simulink model "steering_mpc"  (R2024b)
settings: Solver=VariableStepAuto  StartTime=0  StopTime=84  FixedStep=0.001  RelTol=1e-3  AbsTol=1e-6
values from neighbouring files (symbols this model uses):
  m = 1575    [model.m]
undefined symbols (not defined in the file or in its folder): h, km, MPCController, s, sigbuilder_block
libraries: simulink_extras x6, ctrlSharedLib x2, aerolibconvert2 x2, Solver_SF x1, slpidlib x1
settings Model: Creator=dhall  LastModifiedBy=yassine
settings SolverCC: AlgebraicLoopSolver=TrustRegion
settings DataIOCC: SaveFormat=Array  SignalLoggingSaveFormat=ModelDataLogs  ReturnWorkspaceOutputs=off  SignalLoggingName=sigsOut
settings OptimizationCC: BooleanDataType=off  ReuseModelBlockBuffer=off  InitFltsAndDblsToZero=on
settings DebuggingCC: SaveWithParameterizedLinksMsg=none  UnderspecifiedInitializationDetection=Classic  MergeDetectMultiDrivingBlocksExec=none  SignalResolutionControl=TryResolveAllWithWarning  MultiTaskDSMMsg=warning  MultiTaskCondExecSysMsg=none  UnconnectedInputMsg=warning  UnconnectedOutputMsg=warning  UnconnectedLineMsg=warning
settings HardwareCC: ProdBitPerPointer=32  ProdBitPerSizeT=32  ProdBitPerPtrDiffT=32  ProdLargestAtomicFloat=None  ProdIntDivRoundTo=Undefined  ProdEndianess=Unspecified  ProdWordSize=32  ProdHWDeviceType=32-bit Generic  TargetUnknown=on
settings ModelReferenceCC: EnableRefExpFcnMdlSchedulingChecks=on  PropagateSignalLabelsOutOfModel=off
settings RTWCC: TemplateMakefile=grt_vc.tmf  GPUComputeCapability=3.5  DLArmComputeVersion=19.05
settings GRTTargetCC: TargetFcnLib=ansi_tfl_tmw.mat  TargetLangStandard=C89/C90 (ANSI)  ModelReferenceCompliant=off  CombineOutputUpdateFcns=off  MatFileLogging=off  GRTInterface=on
settings ConfigComp: CovMetricSettings=dw  CovSaveCumulativeToWorkspaceVar=on  CovSaveSingleToWorkspaceVar=on

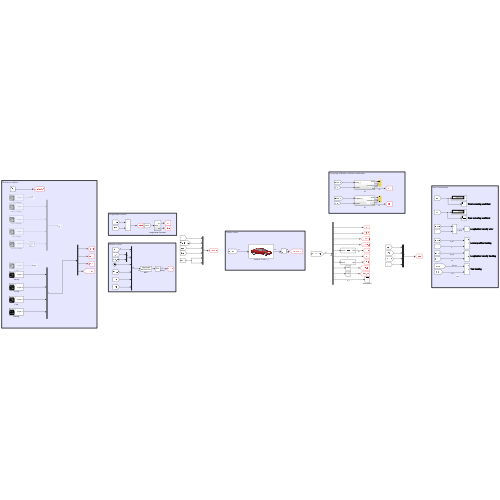
[thumbnail: Simulink's stored preview of the top-level diagram]
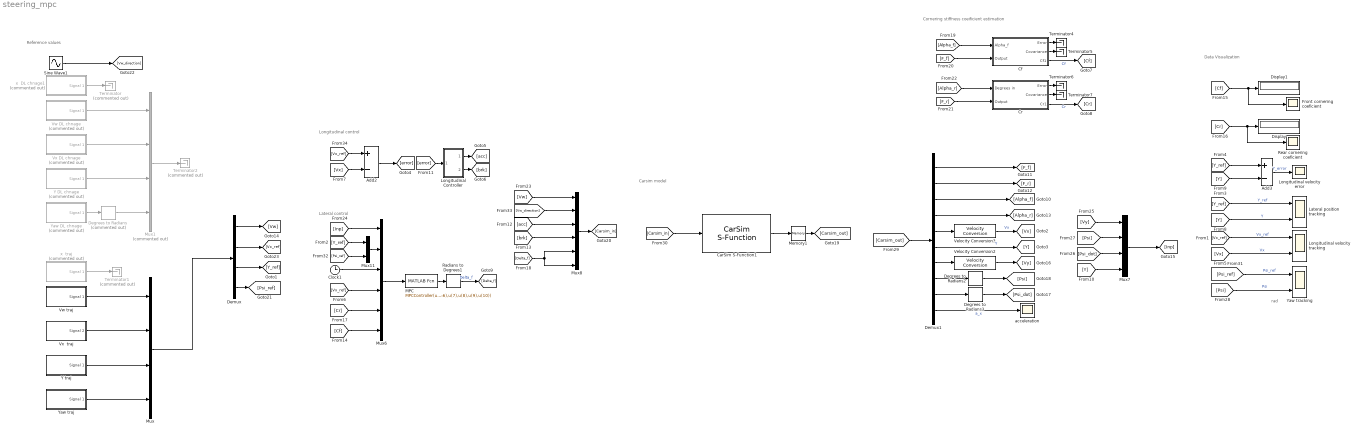
== system steering_mpc ==
  note: Data Visualization
  note: Carsim model
  note: Reference values
  note: Cornering stiffness coeificient estimation
  note: Lateral control
  note: Longitudinal control
  note: rad
  " x  DL chnage1" : Subsystem  Tag=STV Subsys  Commented=on  LoadFcn=sigbuilder_block('load');  StartFcn=sigbuilder_block('start');  StopFcn=sigbuilder_block('stop');  ClipboardFcn=sigbuilder_block('clipboard');  mask(Sigbuilder block){tuvar=[0:10]}
      mask help: Simulink:masks:SigbuilderBlock_MD
      mask init:
      | if ~strcmp(get_param(bdroot(gcbh),'SimulationStatus'),'stopped') tuvar = sigbuilder_block('maskInit'); end
      settings: CopyFcn=sigbuilder_block('copy');  DeleteFcn=sigbuilder_block('delete');  ModelCloseFcn=sigbuilder_block('modelClose');  PreSaveFcn=sigbuilder_block('preSave');  PauseFcn=sigbuilder_block('pause');  ContinueFcn=sigbuilder_block('continue');  NameChangeFcn=sigbuilder_block('namechange');  OpenFcn=sigbuilder_block('open',[474 22.5 1440 689.25 ]);  CloseFcn=sigbuilder_block('close');
      mask Display: plot(0, 0, 100, 100,[2, 2, 32, 32, 2], [68, 8, 8, 68, 68],[32, 2], [38, 38], [32, 19, 2],[53, 60, 44], [32, 17, 17, 2],[16, 16, 31, 31]);txt = getActiveGroup(gcbh);text(2, 100, txt,'verticalAlignment', 'top');
  " x  traj" : Subsystem  Tag=STV Subsys  Commented=on  LoadFcn=sigbuilder_block('load');  StartFcn=sigbuilder_block('start');  StopFcn=sigbuilder_block('stop');  ClipboardFcn=sigbuilder_block('clipboard');  mask(Sigbuilder block){tuvar=[0:10]}
      mask help: Simulink:masks:SigbuilderBlock_MD
      mask init:
      | if ~strcmp(get_param(bdroot(gcbh),'SimulationStatus'),'stopped') tuvar = sigbuilder_block('maskInit'); end
      settings: CopyFcn=sigbuilder_block('copy');  DeleteFcn=sigbuilder_block('delete');  ModelCloseFcn=sigbuilder_block('modelClose');  PreSaveFcn=sigbuilder_block('preSave');  PauseFcn=sigbuilder_block('pause');  ContinueFcn=sigbuilder_block('continue');  NameChangeFcn=sigbuilder_block('namechange');  OpenFcn=sigbuilder_block('open',[65.25 51.75 1440 651.75 ]);  CloseFcn=sigbuilder_block('close');
      mask Display: plot(0, 0, 100, 100,[2, 2, 32, 32, 2], [68, 8, 8, 68, 68],[32, 2], [38, 38], [32, 19, 2],[53, 60, 44], [32, 17, 17, 2],[16, 16, 31, 31]);txt = getActiveGroup(gcbh);text(2, 100, txt,'verticalAlignment', 'top');
  Add2 : Sum  Inputs=+-
  Add3 : Sum  Inputs=+-
  CarSim S-Function1 : Solver_SF/CarSim S-Function  Priority=1  VehicleCode=i_i  SIMFILE=simfile
  Cf : Subsystem
  Clock1 : Clock
  Cr : Subsystem
  Degrees to Radians : simulink_extras/Transformations/Degrees to Radians  Commented=on
  Degrees to Radians2 : simulink_extras/Transformations/Degrees to Radians
  Degrees to Radians3 : simulink_extras/Transformations/Degrees to Radians
  Demux : Demux
  Demux1 : Demux  Outputs=10
  Display : Display
  Display1 : Display
  Front cornering coeficient : Scope
  Lateral position tracking : Scope  NumInputPorts=2
  Longitudinal Controller : Subsystem
  Longitudinal velocity error : Scope
  Longitudinal velocity tracking : Scope  NumInputPorts=2
  MPC : MATLABFcn  MATLABFcn=MPCController(u(1:4),u(5:6),u(7),u(8),u(9),u(10))  SampleTime=0.1
  Memory1 : Memory
  Mux : Mux
  Mux1 : Mux  Commented=on
  Mux11 : Mux  Inputs=2
  Mux6 : Mux  Inputs=6
  Mux7 : Mux
  Mux8 : Mux  Inputs=6
  Radians to Degrees1 : simulink_extras/Transformations/Radians to Degrees
  Rear cornering coeficient : Scope
  Sine Wave1 : Sin  Amplitude=90  Frequency=0.45  SampleTime=0
  Terminator : Terminator  Commented=on
  Terminator1 : Terminator  Commented=on
  Terminator2 : Terminator  Commented=on
  Terminator{4..7} (4 alike) : Terminator
      settings: Tag=Controls_Lib  Description=Terminator  CopyFcn=Lib_CopyFcn(gcb);  PreDeleteFcn=Lib_PreDeleteFcn(gcb);
  Velocity Conversion2 : aerolibconvert2/Velocity Conversion  IU=km/h  OU=m/s
  Velocity Conversion3 : aerolibconvert2/Velocity Conversion  IU=km/h  OU=m/s
  Vw DL chnage : Subsystem  Tag=STV Subsys  Commented=on  LoadFcn=sigbuilder_block('load');  StartFcn=sigbuilder_block('start');  StopFcn=sigbuilder_block('stop');  ClipboardFcn=sigbuilder_block('clipboard');  mask(Sigbuilder block){tuvar=[0:10]}
      mask help: Simulink:masks:SigbuilderBlock_MD
      mask init:
      | if ~strcmp(get_param(bdroot(gcbh),'SimulationStatus'),'stopped') tuvar = sigbuilder_block('maskInit'); end
      settings: CopyFcn=sigbuilder_block('copy');  DeleteFcn=sigbuilder_block('delete');  ModelCloseFcn=sigbuilder_block('modelClose');  PreSaveFcn=sigbuilder_block('preSave');  PauseFcn=sigbuilder_block('pause');  ContinueFcn=sigbuilder_block('continue');  NameChangeFcn=sigbuilder_block('namechange');  OpenFcn=sigbuilder_block('open',[6 38.25 1428 648.75 ]);  CloseFcn=sigbuilder_block('close');
      mask Display: plot(0, 0, 100, 100,[2, 2, 32, 32, 2], [68, 8, 8, 68, 68],[32, 2], [38, 38], [32, 19, 2],[53, 60, 44], [32, 17, 17, 2],[16, 16, 31, 31]);txt = getActiveGroup(gcbh);text(2, 100, txt,'verticalAlignment', 'top');
  Vw traj : Subsystem  Tag=STV Subsys  LoadFcn=sigbuilder_block('load');  StartFcn=sigbuilder_block('start');  StopFcn=sigbuilder_block('stop');  ClipboardFcn=sigbuilder_block('clipboard');  mask(Sigbuilder block){tuvar=[0:10]}
      mask help: Simulink:masks:SigbuilderBlock_MD
      mask init:
      | if ~strcmp(get_param(bdroot(gcbh),'SimulationStatus'),'stopped') tuvar = sigbuilder_block('maskInit'); end
      settings: CopyFcn=sigbuilder_block('copy');  DeleteFcn=sigbuilder_block('delete');  ModelCloseFcn=sigbuilder_block('modelClose');  PreSaveFcn=sigbuilder_block('preSave');  PauseFcn=sigbuilder_block('pause');  ContinueFcn=sigbuilder_block('continue');  NameChangeFcn=sigbuilder_block('namechange');  OpenFcn=sigbuilder_block('open',[195.75 152.25 1428 689.25 ]);  CloseFcn=sigbuilder_block('close');
      mask Display: plot(0, 0, 100, 100,[2, 2, 32, 32, 2], [68, 8, 8, 68, 68],[32, 2], [38, 38], [32, 19, 2],[53, 60, 44], [32, 17, 17, 2],[16, 16, 31, 31]);txt = getActiveGroup(gcbh);text(2, 100, txt,'verticalAlignment', 'top');
  Vx  traj : Subsystem  Tag=STV Subsys  LoadFcn=sigbuilder_block('load');  StartFcn=sigbuilder_block('start');  StopFcn=sigbuilder_block('stop');  ClipboardFcn=sigbuilder_block('clipboard');  mask(Sigbuilder block){tuvar=[0:10]}
      mask help: Simulink:masks:SigbuilderBlock_MD
      mask init:
      | if ~strcmp(get_param(bdroot(gcbh),'SimulationStatus'),'stopped') tuvar = sigbuilder_block('maskInit'); end
      settings: CopyFcn=sigbuilder_block('copy');  DeleteFcn=sigbuilder_block('delete');  ModelCloseFcn=sigbuilder_block('modelClose');  PreSaveFcn=sigbuilder_block('preSave');  PauseFcn=sigbuilder_block('pause');  ContinueFcn=sigbuilder_block('continue');  NameChangeFcn=sigbuilder_block('namechange');  OpenFcn=sigbuilder_block('open',[6 36 1908 945.75 ]);  CloseFcn=sigbuilder_block('close');
      mask Display: plot(0, 0, 100, 100,[2, 2, 32, 32, 2], [68, 8, 8, 68, 68],[32, 2], [38, 38], [32, 19, 2],[53, 60, 44], [32, 17, 17, 2],[16, 16, 31, 31]);txt = getActiveGroup(gcbh);text(2, 100, txt,'verticalAlignment', 'top');
  Vx DL chnage : Subsystem  Tag=STV Subsys  Commented=on  LoadFcn=sigbuilder_block('load');  StartFcn=sigbuilder_block('start');  StopFcn=sigbuilder_block('stop');  ClipboardFcn=sigbuilder_block('clipboard');  mask(Sigbuilder block){tuvar=[0:10]}
      mask help: Simulink:masks:SigbuilderBlock_MD
      mask init:
      | if ~strcmp(get_param(bdroot(gcbh),'SimulationStatus'),'stopped') tuvar = sigbuilder_block('maskInit'); end
      settings: CopyFcn=sigbuilder_block('copy');  DeleteFcn=sigbuilder_block('delete');  ModelCloseFcn=sigbuilder_block('modelClose');  PreSaveFcn=sigbuilder_block('preSave');  PauseFcn=sigbuilder_block('pause');  ContinueFcn=sigbuilder_block('continue');  NameChangeFcn=sigbuilder_block('namechange');  OpenFcn=sigbuilder_block('open',[6 38.25 1428 648.75 ]);  CloseFcn=sigbuilder_block('close');
      mask Display: plot(0, 0, 100, 100,[2, 2, 32, 32, 2], [68, 8, 8, 68, 68],[32, 2], [38, 38], [32, 19, 2],[53, 60, 44], [32, 17, 17, 2],[16, 16, 31, 31]);txt = getActiveGroup(gcbh);text(2, 100, txt,'verticalAlignment', 'top');
  Y DL chnage : Subsystem  Tag=STV Subsys  Commented=on  LoadFcn=sigbuilder_block('load');  StartFcn=sigbuilder_block('start');  StopFcn=sigbuilder_block('stop');  ClipboardFcn=sigbuilder_block('clipboard');  mask(Sigbuilder block){tuvar=[0:10]}
      mask help: Simulink:masks:SigbuilderBlock_MD
      mask init:
      | if ~strcmp(get_param(bdroot(gcbh),'SimulationStatus'),'stopped') tuvar = sigbuilder_block('maskInit'); end
      settings: CopyFcn=sigbuilder_block('copy');  DeleteFcn=sigbuilder_block('delete');  ModelCloseFcn=sigbuilder_block('modelClose');  PreSaveFcn=sigbuilder_block('preSave');  PauseFcn=sigbuilder_block('pause');  ContinueFcn=sigbuilder_block('continue');  NameChangeFcn=sigbuilder_block('namechange');  OpenFcn=sigbuilder_block('open',[6 22.5 1428 689.25 ]);  CloseFcn=sigbuilder_block('close');
      mask Display: plot(0, 0, 100, 100,[2, 2, 32, 32, 2], [68, 8, 8, 68, 68],[32, 2], [38, 38], [32, 19, 2],[53, 60, 44], [32, 17, 17, 2],[16, 16, 31, 31]);txt = getActiveGroup(gcbh);text(2, 100, txt,'verticalAlignment', 'top');
  Y traj : Subsystem  Tag=STV Subsys  LoadFcn=sigbuilder_block('load');  StartFcn=sigbuilder_block('start');  StopFcn=sigbuilder_block('stop');  ClipboardFcn=sigbuilder_block('clipboard');  mask(Sigbuilder block){tuvar=[0:10]}
      mask help: Simulink:masks:SigbuilderBlock_MD
      mask init:
      | if ~strcmp(get_param(bdroot(gcbh),'SimulationStatus'),'stopped') tuvar = sigbuilder_block('maskInit'); end
      settings: CopyFcn=sigbuilder_block('copy');  DeleteFcn=sigbuilder_block('delete');  ModelCloseFcn=sigbuilder_block('modelClose');  PreSaveFcn=sigbuilder_block('preSave');  PauseFcn=sigbuilder_block('pause');  ContinueFcn=sigbuilder_block('continue');  NameChangeFcn=sigbuilder_block('namechange');  OpenFcn=sigbuilder_block('open',[126 246.5 1428 689.5 ]);  CloseFcn=sigbuilder_block('close');
      mask Display: plot(0, 0, 100, 100,[2, 2, 32, 32, 2], [68, 8, 8, 68, 68],[32, 2], [38, 38], [32, 19, 2],[53, 60, 44], [32, 17, 17, 2],[16, 16, 31, 31]);txt = getActiveGroup(gcbh);text(2, 100, txt,'verticalAlignment', 'top');
  Yaw DL chnage : Subsystem  Tag=STV Subsys  Commented=on  LoadFcn=sigbuilder_block('load');  StartFcn=sigbuilder_block('start');  StopFcn=sigbuilder_block('stop');  ClipboardFcn=sigbuilder_block('clipboard');  mask(Sigbuilder block){tuvar=[0:10]}
      mask help: Simulink:masks:SigbuilderBlock_MD
      mask init:
      | if ~strcmp(get_param(bdroot(gcbh),'SimulationStatus'),'stopped') tuvar = sigbuilder_block('maskInit'); end
      settings: CopyFcn=sigbuilder_block('copy');  DeleteFcn=sigbuilder_block('delete');  ModelCloseFcn=sigbuilder_block('modelClose');  PreSaveFcn=sigbuilder_block('preSave');  PauseFcn=sigbuilder_block('pause');  ContinueFcn=sigbuilder_block('continue');  NameChangeFcn=sigbuilder_block('namechange');  OpenFcn=sigbuilder_block('open',[1344.75 109.5 1428 689.25 ]);  CloseFcn=sigbuilder_block('close');
      mask Display: plot(0, 0, 100, 100,[2, 2, 32, 32, 2], [68, 8, 8, 68, 68],[32, 2], [38, 38], [32, 19, 2],[53, 60, 44], [32, 17, 17, 2],[16, 16, 31, 31]);txt = getActiveGroup(gcbh);text(2, 100, txt,'verticalAlignment', 'top');
  Yaw tracking : Scope  NumInputPorts=2
  Yaw traj : Subsystem  Tag=STV Subsys  LoadFcn=sigbuilder_block('load');  StartFcn=sigbuilder_block('start');  StopFcn=sigbuilder_block('stop');  ClipboardFcn=sigbuilder_block('clipboard');  mask(Sigbuilder block){tuvar=[0:10]}
      mask help: Simulink:masks:SigbuilderBlock_MD
      mask init:
      | if ~strcmp(get_param(bdroot(gcbh),'SimulationStatus'),'stopped') tuvar = sigbuilder_block('maskInit'); end
      settings: CopyFcn=sigbuilder_block('copy');  DeleteFcn=sigbuilder_block('delete');  ModelCloseFcn=sigbuilder_block('modelClose');  PreSaveFcn=sigbuilder_block('preSave');  PauseFcn=sigbuilder_block('pause');  ContinueFcn=sigbuilder_block('continue');  NameChangeFcn=sigbuilder_block('namechange');  OpenFcn=sigbuilder_block('open',[6 36 1908 945.75 ]);  CloseFcn=sigbuilder_block('close');
      mask Display: plot(0, 0, 100, 100,[2, 2, 32, 32, 2], [68, 8, 8, 68, 68],[32, 2], [38, 38], [32, 19, 2],[53, 60, 44], [32, 17, 17, 2],[16, 16, 31, 31]);txt = getActiveGroup(gcbh);text(2, 100, txt,'verticalAlignment', 'top');
  acceleration : Scope
  wires:
  Demux1/1 -> [F_f]
  Demux1/8 -> Degrees to Radians2/1
  Degrees to Radians2/1 -> [Psi]
  MPC/1 -> Radians to Degrees1/1
  Add2/1 -> [error]
  [acc] -> Mux8/3
  Demux1/9 -> Degrees to Radians3/1
  Velocity Conversion2/1 -> [Vy]
  Add3/1 -> Longitudinal velocity error/1  "Y_error"
  Demux1/5 -> Velocity Conversion3/1
  Degrees to Radians3/1 -> [Psi_dot]
  [Carsim_out] -> Demux1/1
  CarSim S-Function1/1 -> Memory1/1
  Clock1/1 -> Mux6/3
  Demux1/7 -> Velocity Conversion2/1
  [Carsim_in] -> CarSim S-Function1/1
  Mux11/1 -> Mux6/2
  Demux1/3 -> [Alpha_f]
  Sine Wave1/1 -> [Vw_direction]
  " x  DL chnage1"/1(Signal 1) -> Terminator/1
  " x  traj"/1(Signal 1) -> Terminator1/1
  [Psi_ref] -> Yaw tracking/1  "Psi_ref"
  [Vx_ref] -> Add2/1
  Demux1/10 -> acceleration/1  "a_x"
  Vx DL chnage/1(Signal 1) -> Mux1/2
  Vx  traj/1(Signal 2) -> Mux/2
  [Vx_ref] -> Longitudinal velocity tracking/1  "Vx_ref"
  Y DL chnage/1(Signal 1) -> Mux1/3
  Y traj/1(Signal 1) -> Mux/3
  [Y_ref] -> Lateral position tracking/1  "Y_ref"
  [Y_ref] -> Add3/1
  [Vx] -> Longitudinal velocity tracking/2  "Vx"
  Velocity Conversion3/1 -> [Vx]  "Vx"
  [Vx] -> Add2/2
  [Y] -> Add3/2
  Demux1/6 -> [Y]  "Y"
  [Y] -> Lateral position tracking/2  "Y"
  [error] -> Longitudinal Controller/1(error)
  Longitudinal Controller/1(acc) -> [acc]
  Longitudinal Controller/2(brk) -> [brk]
  Cf/3(Cf1) -> [Cf]  "Cf"
  [Cf] -> Display1/1, Front cornering coeficient/1
  Cf/1(Error) -> Terminator4/1
  Cf/2(Covariance) -> Terminator5/1
  Cr/3(Cr1) -> [Cr]  "Cr"
  [Cr] -> Rear cornering coeficient/1, Display/1
  Cr/1(Error) -> Terminator6/1
  Cr/2(Covariance) -> Terminator7/1
  Radians to Degrees1/1 -> [Delta_f]  "Delta_f"
  [Alpha_f] -> Cf/1(Alpha_f)
  [F_f] -> Cf/2(Output)
  Demux1/2 -> [F_r]
  [F_r] -> Cr/2(Output)
  Demux1/4 -> [Alpha_r]
  [Alpha_r] -> Cr/1(Degrees in)
  Vw traj/1(Signal 1) -> Mux/1
  [Psi] -> Yaw tracking/2  "Psi"
  Memory1/1 -> [Carsim_out]
  Mux8/1 -> [Carsim_in]
  Vw DL chnage/1(Signal 1) -> Mux1/1
  [Psi_ref] -> Mux11/2
  Yaw DL chnage/1(Signal 1) -> Degrees to Radians/1
  Degrees to Radians/1 -> Mux1/4
  [Vw_direction] -> Mux8/2
  Mux7/1 -> [Inp]
  [Psi] -> Mux7/2
  [Y] -> Mux7/4
  [Vy] -> Mux7/1
  [Psi_dot] -> Mux7/3
  [Cr] -> Mux6/5
  [Cf] -> Mux6/6
  [Inp] -> Mux6/1
  [Vx_ref] -> Mux6/4
  [Delta_f] -> Mux8/6, Mux8/5
  [brk] -> Mux8/4
  [Y_ref] -> Mux11/1
  Mux6/1 -> MPC/1
  [Vw] -> Mux8/1
  Yaw traj/1(Signal 1) -> Mux/4
  Demux/1 -> [Vw]
  Demux/2 -> [Vx_ref]
  Demux/3 -> [Y_ref]
  Demux/4 -> [Psi_ref]
  Mux1/1 -> Terminator2/1
  Mux/1 -> Demux/1

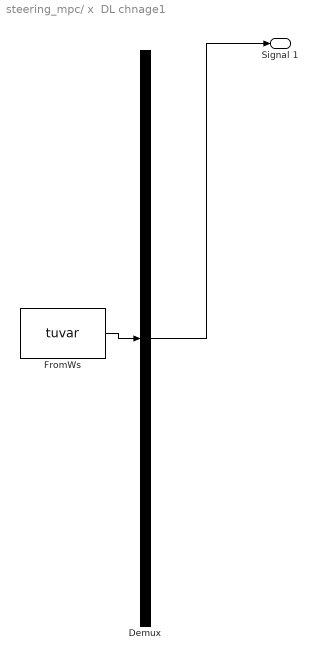
== system steering_mpc/ x  DL chnage1 ==
  Demux : Demux  Tag=STV Demux  Outputs=1
      settings: DisplayOption=none
  FromWs : FromWorkspace  Tag=STV FromWs  VariableName=tuvar
      SigBuilderData=|
      | common.afterFinalStr = 'Extrapolate'
      | common.sampleTime = 0
      | dataSet.timeRange = [0 8.6]
      | dataSet.name = 'Group 1'
      | sbobj.Groups.Name = 'Group 1'
      | sbobj.Groups.Signals.Name = 'Signal 1'
      | sbobj.Groups.Signals.XData = [0 0.1 0.2 0.3 0.4 0.5 0.6 0.7 0.8 0.9 1 1.1 1.2 1.3 1.4 1.5 1.6 1.7 1.8 1.9 2 2.1 2.2 2.3 2.4 2.5 2.6 2.7 2.8 2.9 3 3.1 3.2 3.3 3.4 3.5 3.6 3.7 3.8 3.9 4 4.1 4.2 4.3 4.4 4.5 4.6 4.7 4.8 4.9 5 5.1 5.2 5.3 5.4 5.5 5.6 5.7 5.8 5.9 6 6.1 6.2 6.3 6.4 6.5 6.6 6.7 6.8 6.9 7 7.1 7.2 7.3 7.4 7.5 7.6 7.7 7.8 7.9 8 8.1 8.2 8.3 8.4 8.5 8.6 8.6]
      | sbobj.Groups.Signals.YData = [0 1.40382369215 2.81533103222 4.23452088579 5.6614062982 7.10044825923 8.55471249429 10.023188748 11.5050859453 13.002763305 14.5182223781 16.0437367688 17.5723178537 19.1036308309 20.6404977369 22.1850981616 23.7369352904 25.29540146 26.8607578328 28.4360381847 30.0225679659 31.6217163445 33.2332823068 34.8554095816 36.4886582653 38.1335016448 39.7902907389 41.4610263852 43.1461724696 44.8451392514 46.5573608906 48.2841741387 50.0272574966 51.7859299951 53.5577743918 55.3391017968 57.1298579812 58.9304850779 60.7409740716 62.5491088271 64.3499140704 66.1429390646 67.92766822 69.7041107991 71.4732732494 73.2360892249 74.9935040841 76.7463517639 78.4935117684 80.2332444025 81.9648406428 83.6876845274 85.4014121891 87.1074509704 88.8064894172 90.4989743473 92.18534608 93.8660019215 95.5409908601 97.2071549746 98.8631569055 100.508605984 102.143156505 103.766359581 105.377983513 106.978450273 108.568157717 110.147567014 111.718956488 113.282766249 114.838783539 116.38685481 117.927256016 119.462559204 120.993231574 122.519248333 124.040591782 125.557250039 127.069215807 128.576485189 130.079056569 131.579061817 133.079061815 134.579061815 136.079061815 137.579061813 139.079061812 139.079061812]
      | sbobj.Groups.TimeRange = [0 8.6]
  Signal 1 : Outport  Tag=STV Outport
  wires:
  FromWs/1 -> Demux/1
  Demux/1 -> Signal 1/1

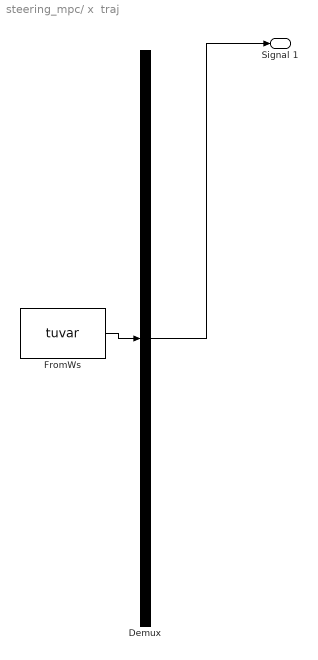
== system steering_mpc/ x  traj ==
  Demux : Demux  Tag=STV Demux  Outputs=1
      settings: DisplayOption=none
  FromWs : FromWorkspace  Tag=STV FromWs  VariableName=tuvar
      SigBuilderData=|
      | common.afterFinalStr = 'Extrapolate'
      | common.sampleTime = 0
      | dataSet.timeRange = [0 84.64]
      | dataSet.name = 'Group 1'
      | sbobj.Groups.Name = 'Group 1'
      | sbobj.Groups.Signals.Name = 'Signal 1'
      | sbobj.Groups.Signals.XData = [0 0.23 0.46 0.69 0.92 1.15 1.38 1.61 1.84 2.07 2.3 2.53 ... (369 elements, 1x369)]
      | sbobj.Groups.Signals.YData = [0.65 0.146763834666 -0.364544706871 -0.883930779874 -1.41139991584 -1.94695797534 -2.49061108836 -3.04236558063 -3.60222788482 -4.17020443488 -4.74630154209 -5.33052525115 ... (369 elements, 1x369)]
      | sbobj.Groups.TimeRange = [0 84.64]
  Signal 1 : Outport  Tag=STV Outport
  wires:
  FromWs/1 -> Demux/1
  Demux/1 -> Signal 1/1

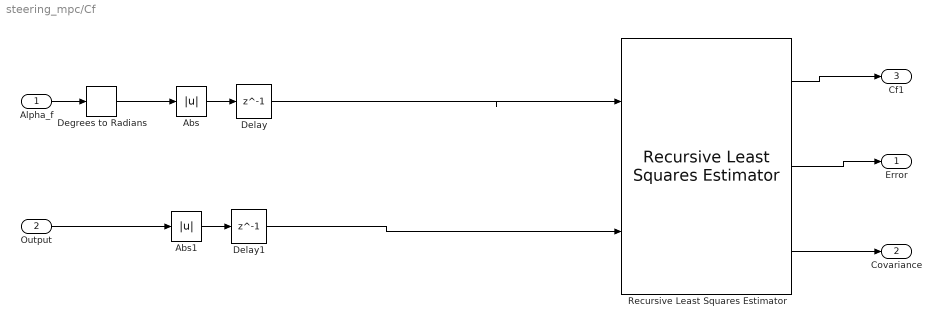
== system steering_mpc/Cf ==
  Alpha_f : Inport
  Output : Inport  Port=2
  Abs : Abs  SaturateOnIntegerOverflow=off
  Abs1 : Abs  SaturateOnIntegerOverflow=off
  Degrees to Radians : simulink_extras/Transformations/Degrees to Radians
  Delay : Delay  DelayLength=1
  Delay1 : Delay  DelayLength=1
  Recursive Least Squares Estimator : ctrlSharedLib/Recursive Least Squares Estimator  InitialEstimateSource=None  InitialParameterData=1  P0=1e4  InitialRegressors=0  InitialOutputs=0  History=Infinite  WindowLength=200  EstimationMethod=Forgetting Factor  AdaptationParameter=1-3e-4  HasTimeVaryingAdaptationParameter=off  NormalizationBias=eps  OutputError=on  OutputP=on  AddEnablePort=off  InputProcessing=Sample-based  Ts=-1
  Error : Outport
  Covariance : Outport  Port=2
  Cf1 : Outport  Port=3
  wires:
  Alpha_f/1 -> Degrees to Radians/1
  Degrees to Radians/1 -> Abs/1
  Output/1 -> Abs1/1
  Delay/1 -> Recursive Least Squares Estimator/1
  Delay1/1 -> Recursive Least Squares Estimator/2
  Recursive Least Squares Estimator/1 -> Cf1/1
  Recursive Least Squares Estimator/3 -> Covariance/1
  Recursive Least Squares Estimator/2 -> Error/1
  Abs/1 -> Delay/1
  Abs1/1 -> Delay1/1

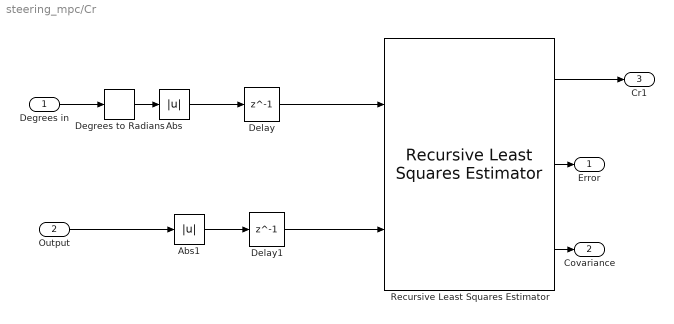
== system steering_mpc/Cr ==
  Degrees in : Inport
  Output : Inport  Port=2
  Abs : Abs  SaturateOnIntegerOverflow=off
  Abs1 : Abs  SaturateOnIntegerOverflow=off
  Degrees to Radians : simulink_extras/Transformations/Degrees to Radians
  Delay : Delay  DelayLength=1
  Delay1 : Delay  DelayLength=1
  Recursive Least Squares Estimator : ctrlSharedLib/Recursive Least Squares Estimator  InitialEstimateSource=None  InitialParameterData=1  P0=1e4  InitialRegressors=0  InitialOutputs=0  History=Infinite  WindowLength=200  EstimationMethod=Forgetting Factor  AdaptationParameter=1-3e-4  HasTimeVaryingAdaptationParameter=off  NormalizationBias=eps  OutputError=on  OutputP=on  AddEnablePort=off  InputProcessing=Sample-based  Ts=-1
  Error : Outport
  Covariance : Outport  Port=2
  Cr1 : Outport  Port=3
  wires:
  Recursive Least Squares Estimator/1 -> Cr1/1
  Recursive Least Squares Estimator/3 -> Covariance/1
  Recursive Least Squares Estimator/2 -> Error/1
  Delay/1 -> Recursive Least Squares Estimator/1
  Delay1/1 -> Recursive Least Squares Estimator/2
  Degrees in/1 -> Degrees to Radians/1
  Abs/1 -> Delay/1
  Abs1/1 -> Delay1/1
  Degrees to Radians/1 -> Abs/1
  Output/1 -> Abs1/1

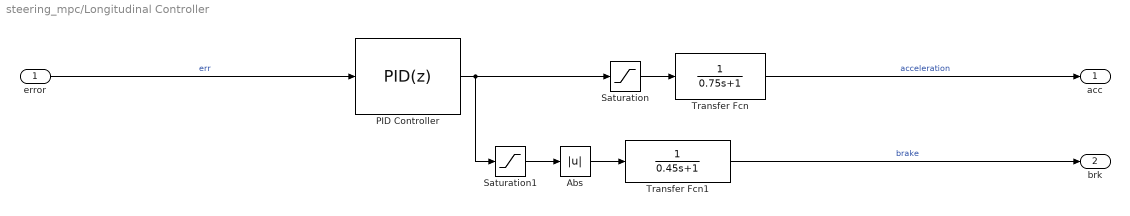
== system steering_mpc/Longitudinal Controller ==
  error : Inport
  Abs : Abs  SaturateOnIntegerOverflow=off
  PID Controller : slpidlib/PID Controller  Controller=PID  Form=Parallel  TimeDomain=Discrete-time  UseExternalTs=off  SampleTime=-1  IntegratorMethod=Forward Euler  FilterMethod=Forward Euler  ControllerParametersSource=internal  P=5.52  I=0.0547  UseKiTs=off  D=0.469  UseExternalDerivativeSource=off  N=100  UseFilter=off  TunerSelectOption=Transfer Function Based (PID Tuner App)  InitialConditionSource=internal  InitialConditionForIntegrator=0  InitialConditionForFilter=0  DifferentiatorICPrevScaledInput=0  ExternalReset=none  TrackingMode=off  Kt=1  LimitOutput=off  SatLimitsSource=internal  UpperSaturationLimit=inf  LowerSaturationLimit=-inf  LinearizeAsGain=on  AntiWindupMode=none  Kb=1  LimitIntegrator=off  UpperIntegratorSaturationLimit=inf  LowerIntegratorSaturationLimit=-inf  POutMin=[]  POutMax=[]  IOutMin=[]  IOutMax=[]  DOutMin=[]  DOutMax=[]  NOutMin=[]  NOutMax=[]  SumOutMin=[]  SumOutMax=[]  SaturationOutMin=[]  SaturationOutMax=[]  PParamMin=[]  PParamMax=[]  IParamMin=[]  IParamMax=[]  DParamMin=[]  DParamMax=[]  NParamMin=[]  NParamMax=[]  KbParamMin=[]  KbParamMax=[]  KtParamMin=[]  KtParamMax=[]  KbOutMin=[]  KbOutMax=[]  KtOutMin=[]  KtOutMax=[]  IntegratorOutMin=[]  IntegratorOutMax=[]  FilterOutMin=[]  FilterOutMax=[]  SumI1OutMin=[]  SumI1OutMax=[]  SumI2OutMin=[]  SumI2OutMax=[]  SumI3OutMin=[]  SumI3OutMax=[]  SumI4OutMin=[]  SumI4OutMax=[]  SumDOutMin=[]  SumDOutMax=[]  DifferentiatorOutMin=[]  DifferentiatorOutMax=[]  FilterDiffOutCoefMin=[]  FilterDiffOutCoefMax=[]  ReciprocalOutMin=[]  ReciprocalOutMax=[]  SumDenOutMin=[]  SumDenOutMax=[]  SumNumOutMin=[]  SumNumOutMax=[]  DivideOutMin=[]  DivideOutMax=[]  UdiffTsProdOutMin=[]  UdiffTsProdOutMax=[]  NTsProdOutMin=[]  NTsProdOutMax=[]  UintegralTsProdOutMin=[]  UintegralTsProdOutMax=[]  UngainTsProdOutMin=[]  UngainTsProdOutMax=[]  ClampingZeroOutDataTypeStr=Inherit: Inherit via back propagation  ClampingZeroOutMin=[]  ClampingZeroOutMax=[]  FilterDenConstantOutDataTypeStr=Inherit: Inherit via back propagation  FilterDenConstantOutMin=[]  FilterDenConstantOutMax=[]  PCopyOutDataTypeStr=Inherit: Inherit via back propagation  PCopyOutMin=[]  PCopyOutMax=[]  NCopyOutDataTypeStr=Inherit: Inherit via back propagation  NCopyOutMin=[]  NCopyOutMax=[]  IntegratorContinuousStateAttributes=''  IntegratorStateMustResolveToSignalObject=off  IntegratorRTWStateStorageClass=Auto  FilterContinuousStateAttributes=''  FilterStateMustResolveToSignalObject=off  FilterRTWStateStorageClass=Auto  ParallelPVariant=InternalParameters  IdealPVariant=Disabled  IVariant=InternalParameters  DVariant=InternalParameters  IntegratorVariant=Discrete  SatVariant=Disabled  AWVariant=Passthrough  PCopyVariant=Disabled  TRVariant=Disabled  FdbkBlocksVariant=Forward  IdealPFdbkVariant=Disabled  SatFdbkVariant=Disabled  DerivativeFilterVariant=Differentiator  NVariant=Passthrough  NCopyVariant=Disabled_SignalSpec  FilterICVariant=InternalICsDifferentiator  IntegratorICVariant=InternalICs  ExternalResetVariant=Disabled  TRSumVariant=Passthrough  SumFdbkVariant=Disabled  SumVariant=Sum_PID  TsampFilterVariant=InternalTs  TsampNgainVariant=Passthrough  TsampIntegralVariant=Disabled_SignalSpec  ExternalSaturationOutDataTypeStr=Inherit: Same as second input  DerivativeSourceVariant=ErrorSignal  PreIntVariant=InternalPreInt
  Saturation : Saturate  UpperLimit=1  LowerLimit=0
  Saturation1 : Saturate  UpperLimit=0  LowerLimit=-5
  Transfer Fcn : TransferFcn  Denominator=[0.75 1]
  Transfer Fcn1 : TransferFcn  Denominator=[0.45 1]
  acc : Outport
  brk : Outport  Port=2
  wires:
  Transfer Fcn/1 -> acc/1  "acceleration"
  PID Controller/1 -> Saturation1/1, Saturation/1
  error/1 -> PID Controller/1  "err"
  Saturation1/1 -> Abs/1
  Abs/1 -> Transfer Fcn1/1
  Saturation/1 -> Transfer Fcn/1
  Transfer Fcn1/1 -> brk/1  "brake"

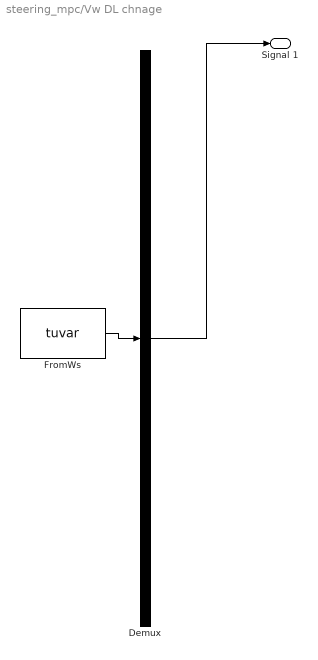
== system steering_mpc/Vw DL chnage ==
  Demux : Demux  Tag=STV Demux  Outputs=1
      settings: DisplayOption=none
  FromWs : FromWorkspace  Tag=STV FromWs  VariableName=tuvar
      SigBuilderData=|
      | common.afterFinalStr = 'Extrapolate'
      | common.sampleTime = 0
      | dataSet.timeRange = [0 8.6]
      | dataSet.name = 'Group 1'
      | sbobj.Groups.Name = 'Group 1'
      | sbobj.Groups.Signals.Name = 'Signal 1'
      | sbobj.Groups.Signals.XData = [0 0.1 0.2 0.2 0.3 0.4 0.5 0.6 0.7 0.8 0.9 1 1.1 1.2 1.3 1.4 1.5 1.6 1.7 1.8 1.9 2 2.1 2.2 2.3 2.4 2.5 2.6 2.6 2.7 2.7 2.8 2.9 3 3.1 3.2 3.3 3.4 3.5 3.6 3.7 3.8 3.9 4 4.1 4.2 4.3 4.4 4.5 4.6 4.7 4.8 4.9 5 5.1 5.2 5.3 5.4 5.5 5.6 5.7 5.8 5.9 6 6.1 6.2 6.3 6.4 6.5 6.6 6.7 6.8 6.9 7 7.1 7.1 7.2 7.3 7.4 7.5 7.6 7.7 7.8 7.9 8 8.1 8.2 8.3 8.4 8.5 8.6]
      | sbobj.Groups.Signals.YData = [19.6 24.4 32.7 32.5 36.4 38.8 40.4 47.1 50.3 51.9 53.2 54.2 54.6 54.6 54.2 53.2 50.9 50.1 48.5 47.7 48 47.8 48.5 49.4 50.5 50.9 51.3 51.1 51.2 50.4 50.3 49.1 45.4 42.1 40.9 39.6 39.7 39.4 38 35.9 35.1 34.2 32.1 30.2 29.1 28.7 29 29.9 30.7 31.8 32.8 34.3 34.9 35 35.7 37.2 37.8 38.9 39.5 39.5 39.5 39.1 38.2 35.9 33.6 30.7 29.3 28.6 27.2 26.3 26.3 26.5 27.4 29.3 29.8 29.7 29.8 30.7 31 33 33.9 34.4 33.9 33.3 32.2 31.1 28 25 23.5 22.7 22.4]
      | sbobj.Groups.TimeRange = [0 8.6]
  Signal 1 : Outport  Tag=STV Outport
  wires:
  FromWs/1 -> Demux/1
  Demux/1 -> Signal 1/1

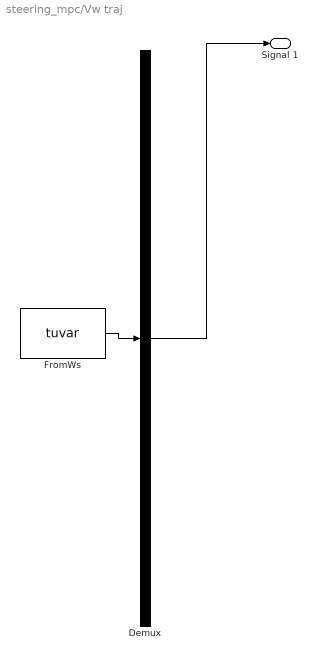
== system steering_mpc/Vw traj ==
  Demux : Demux  Tag=STV Demux  Outputs=1
      settings: DisplayOption=none
  FromWs : FromWorkspace  Tag=STV FromWs  VariableName=tuvar
      SigBuilderData=|
      | common.afterFinalStr = 'Extrapolate'
      | common.sampleTime = 0
      | dataSet.timeRange = [0 84.64]
      | dataSet.name = 'Group 1'
      | sbobj.Groups.Name = 'Group 1'
      | sbobj.Groups.Signals.Name = 'Signal 1'
      | sbobj.Groups.Signals.XData = [0 0.23 0.46 0.69 0.92 1.15 1.38 1.61 1.84 2.07 2.3 2.53 ... (369 elements, 1x369)]
      | sbobj.Groups.Signals.YData = [27.1 27.353 27.606 27.859 28.112 28.5 28.96 29.42 29.88 30.541 31.99 33.439 ... (369 elements, 1x369)]
      | sbobj.Groups.TimeRange = [0 84.64]
  Signal 1 : Outport  Tag=STV Outport
  wires:
  FromWs/1 -> Demux/1
  Demux/1 -> Signal 1/1

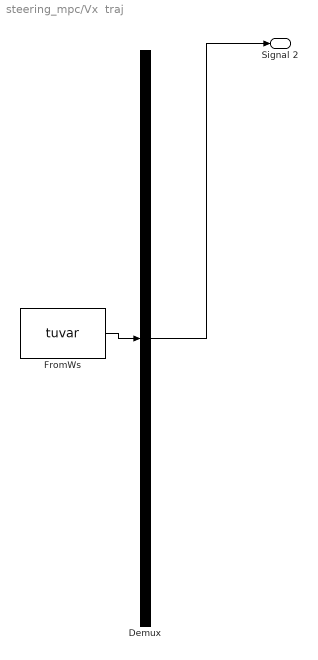
== system steering_mpc/Vx  traj ==
  Demux : Demux  Tag=STV Demux  Outputs=1
      settings: DisplayOption=none
  FromWs : FromWorkspace  Tag=STV FromWs  VariableName=tuvar
      SigBuilderData=|
      | common.afterFinalStr = 'Extrapolate'
      | common.sampleTime = 0
      | dataSet.timeRange = [0 84.64]
      | dataSet.name = 'Group 1'
      | sbobj.Groups.Name = 'Group 1'
      | sbobj.Groups.Signals.Name = 'Signal 2'
      | sbobj.Groups.Signals.XData = [0 0.23 0.46 0.69 0.92 1.15 1.38 1.61 1.84 2.07 2.3 2.53 ... (369 elements, 1x369)]
      | sbobj.Groups.Signals.YData = [0.05 0.7 1.15 1.55 2 2.65 3.25 3.95 4.45 4.9 5.15 5.4 ... (369 elements, 1x369)]
      | sbobj.Groups.TimeRange = [0 84.64]
  Signal 2 : Outport  Tag=STV Outport
  wires:
  FromWs/1 -> Demux/1
  Demux/1 -> Signal 2/1

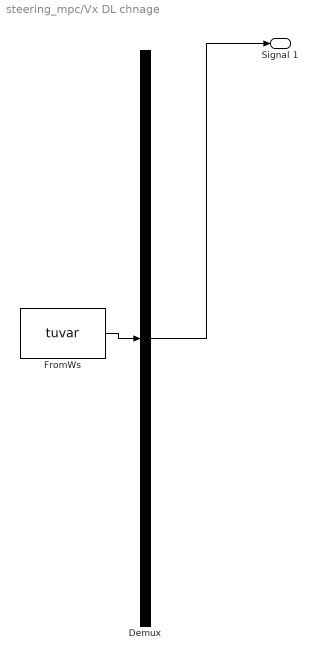
== system steering_mpc/Vx DL chnage ==
  Demux : Demux  Tag=STV Demux  Outputs=1
      settings: DisplayOption=none
  FromWs : FromWorkspace  Tag=STV FromWs  VariableName=tuvar
      SigBuilderData=|
      | common.afterFinalStr = 'Extrapolate'
      | common.sampleTime = 0
      | dataSet.timeRange = [0 8.6]
      | dataSet.name = 'Group 1'
      | sbobj.Groups.Name = 'Group 1'
      | sbobj.Groups.Signals.Name = 'Signal 1'
      | sbobj.Groups.Signals.XData = [0 0.1 0.2 0.3 0.4 0.5 0.6 0.7 0.8 0.9 1 1.1 1.2 1.3 1.4 1.5 1.6 1.7 1.8 1.9 2 2.1 2.2 2.3 2.4 2.5 2.6 2.7 2.8 2.9 3 3.1 3.2 3.3 3.4 3.5 3.6 3.7 3.8 3.9 4 4.1 4.2 4.3 4.4 4.5 4.6 4.7 4.8 4.9 5 5.1 5.2 5.3 5.4 5.5 5.6 5.7 5.8 5.9 6 6.1 6.2 6.3 6.4 6.5 6.6 6.7 6.8 6.9 7 7.1 7.2 7.3 7.4 7.5 7.6 7.7 7.8 7.9 8 8.1 8.2 8.3 8.4 8.5 8.6]
      | sbobj.Groups.Signals.YData = [14 14.0440550225 14.115358608 14.2064929121 14.3101549156 14.45 14.6 14.7689890985 14.9298612177 15.11 15.28 15.43 15.57 15.705926856 15.83 15.95 16.06 16.16 16.24 16.35 16.4450804231 16.5806076226 16.7096359472 16.8368553272 16.9642003593 17.093568143 17.2273955873 17.3786082804 17.5376271666 17.6839795308 17.7963308107 17.8836695471 17.959373843 17.9987537498 18 18 18 18 17.9993390048 17.9875457651 17.964341131 17.9340228274 17.9007917312 17.8592846609 17.8034563926 17.7377441012 17.6665014179 17.5939214982 17.5130240928 17.4224039016 17.3296218562 17.2420174684 17.166097611 17.1005009277 17.0404876364 16.9816688223 16.9197553024 16.8505566704 16.7696004365 16.671748601 16.5617024302 16.4459508882 16.3307376588 16.2169922998 16.0976752186 15.9788998844 15.8672392559 15.768121736 15.6752469369 15.5874236439 15.5065212375 15.4343483282 15.3709385287 15.3066024005 15.2418993934 15.1796445936 15.122601324 15.0734815415 15.0349462339 15.0096058149 15.0000205181 15 15 15 15 15 15]
      | sbobj.Groups.TimeRange = [0 8.6]
  Signal 1 : Outport  Tag=STV Outport
  wires:
  FromWs/1 -> Demux/1
  Demux/1 -> Signal 1/1

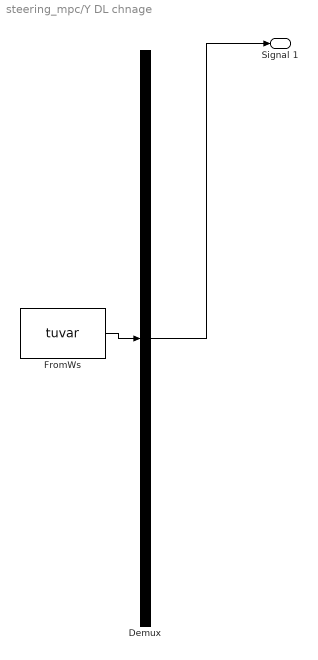
== system steering_mpc/Y DL chnage ==
  Demux : Demux  Tag=STV Demux  Outputs=1
      settings: DisplayOption=none
  FromWs : FromWorkspace  Tag=STV FromWs  VariableName=tuvar
      SigBuilderData=|
      | common.afterFinalStr = 'Extrapolate'
      | common.sampleTime = 0
      | dataSet.timeRange = [0 8.6]
      | dataSet.name = 'Group 1'
      | sbobj.Groups.Name = 'Group 1'
      | sbobj.Groups.Signals.Name = 'Signal 1'
      | sbobj.Groups.Signals.XData = [0 0.1 0.2 0.3 0.4 0.5 0.6 0.7 0.8 0.9 1 1.1 1.2 1.3 1.4 1.5 1.6 1.7 1.8 1.8 1.9 1.9 2 2.1 2.2 2.3 2.4 2.5 2.6 2.7 2.8 2.9 3 3.1 3.2 3.3 3.4 3.5 3.6 3.7 3.8 3.9 4 4.1 4.2 4.3 4.4 4.5 4.6 4.7 4.8 4.9 5 5.1 5.2 5.3 5.4 5.5 5.6 5.7 5.8 5.9 6 6.1 6.2 6.3 6.4 6.5 6.6 6.7 6.8 6.9 7 7.1 7.2 7.3 7.4 7.5 7.6 7.7 7.8 7.9 8 8.1 8.2 8.3 8.4 8.5 8.6 8.6]
      | sbobj.Groups.Signals.YData = [0 0.006 0.012 0.023046 0.037 0.04 0.05 0.08 0.13 0.2 0.31 0.42 0.57 0.72 0.87 1.04 1.23 1.4 1.61 1.62 1.84 1.83 2.08 2.33 2.56 2.88 3.15 3.42 3.63 3.83 3.96 4.06 4.16 4.22 4.22 4.19 4.16 4.06 3.93 3.77 3.62 3.4745782615 3.31818687289 3.15304669643 2.97444845326 2.77979798164 2.57525569105 2.36921320407 2.16988721809 1.98533308829 1.82031921249 1.66932129015 1.52489980491 1.37982547849 1.22726303684 1.06577325472 0.89981188723 0.734043919743 0.573027853144 0.421220174721 0.282928438031 0.15885012028 0.0440566030867 -0.0667029365953 -0.178481773128 -0.29542011902 -0.414879860075 -0.530766422783 -0.637202805923 -0.728617729197 -0.802713116871 -0.861684506097 -0.908012332679 -0.944107574551 -0.972294219774 -0.994216587334 -1.0107321777 -1.02263872501 -1.03072013009 -1.03574652124 -1.0384743298 -1.03964637725 -1.03999197046 -1.04012720351 -1.04019778678 -1.04021503206 -1.04019023828 -1.04013470437 -1.04005972924 -1.04005972924]
      | sbobj.Groups.TimeRange = [0 8.6]
  Signal 1 : Outport  Tag=STV Outport
  wires:
  Demux/1 -> Signal 1/1
  FromWs/1 -> Demux/1

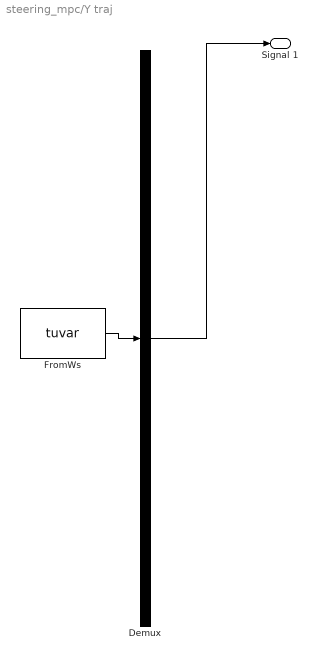
== system steering_mpc/Y traj ==
  Demux : Demux  Tag=STV Demux  Outputs=1
      settings: DisplayOption=none
  FromWs : FromWorkspace  Tag=STV FromWs  VariableName=tuvar
      SigBuilderData=|
      | common.afterFinalStr = 'Extrapolate'
      | common.sampleTime = 0
      | dataSet.timeRange = [0 84.64]
      | dataSet.name = 'Group 1'
      | sbobj.Groups.Name = 'Group 1'
      | sbobj.Groups.Signals.Name = 'Signal 1'
      | sbobj.Groups.Signals.XData = [0 0.23 0.46 0.69 0.92 1.15 1.38 1.61 1.84 2.07 2.3 2.53 ... (369 elements, 1x369)]
      | sbobj.Groups.Signals.YData = [0.06 0.0884593586099 0.117290517342 0.146401376833 0.175691431192 0.20505143814 0.234363083527 0.263498640262 0.292320621708 0.320681429626 0.348422996794 0.37537642446 ... (369 elements, 1x369)]
      | sbobj.Groups.TimeRange = [0 84.64]
  Signal 1 : Outport  Tag=STV Outport
  wires:
  FromWs/1 -> Demux/1
  Demux/1 -> Signal 1/1

== system steering_mpc/Yaw DL chnage ==
  Demux : Demux  Tag=STV Demux  Outputs=1
      settings: DisplayOption=none
  FromWs : FromWorkspace  Tag=STV FromWs  VariableName=tuvar
      SigBuilderData=|
      | common.afterFinalStr = 'Extrapolate'
      | common.sampleTime = 0
      | dataSet.timeRange = [0 8.6]
      | dataSet.name = 'Group 1'
      | sbobj.Groups.Name = 'Group 1'
      | sbobj.Groups.Signals.Name = 'Signal 1'
      | sbobj.Groups.Signals.XData = [0 0.1 0.2 0.3 0.4 0.5 0.6 0.7 0.8 0.9 1 1.1 1.2 1.3 1.4 1.5 1.6 1.7 1.8 1.9 2 2.1 2.2 2.3 2.4 2.5 2.6 2.7 2.8 2.9 3 3.1 3.2 3.3 3.4 3.5 3.6 3.7 3.8 3.9 4 4.1 4.2 4.3 4.4 4.5 4.6 4.7 4.8 4.9 5 5.1 5.2 5.3 5.4 5.5 5.6 5.7 5.8 5.9 6 6.1 6.2 6.3 6.4 6.5 6.6 6.7 6.8 6.9 7 7.1 7.2 7.3 7.4 7.5 7.6 7.7 7.8 7.9 8 8.1 8.2 8.3 8.4 8.5 8.6 8.6]
      | sbobj.Groups.Signals.YData = [0.273191117862 0.35 0.35 0.35 0.45 0.8 1.41591852383 2.35 3.3 3.9 4.6 5.05 5.41123164015 5.70950446367 6.1283990888 6.65987373252 7.30588163843 8.06838756712 8.85141510872 9.35857445024 9.56278465756 9.45655418311 9.08981450662 8.55711497383 7.85762290414 6.98876852712 5.9518543751 4.87475817261 3.820928089 2.79101165106 1.78566090276 0.746841291923 -0.396019426572 -1.64562914651 -2.87324064669 -3.81093373672 -4.44539651513 -4.77090376114 -4.80068398439 -4.8657390232 -5.08713608574 -5.46306785024 -5.99173396147 -6.46942735422 -6.67563393708 -6.61301712749 -6.28435098223 -5.69417589811 -5.13712027875 -4.82393610895 -4.75104222254 -4.91487522675 -5.26906618094 -5.51945298798 -5.61236996213 -5.54961284344 -5.33297049106 -4.96422488327 -4.46600270289 -4.08185757685 -3.87853146605 -3.85255353489 -4.00047553804 -4.21597318548 -4.22619775656 -4.02091036619 -3.60468145863 -2.99834680346 -2.41498084257 -1.91809913142 -1.50639094401 -1.17855243582 -0.927584454561 -0.713262364409 -0.527798489184 -0.370933537345 -0.242409013205 -0.141967216939 -0.0693512445746 -0.0243049880013 -0.0065731349642 -0.0038586248751 -0.00160547049835 0.000216096821645 0.00160607708487 0.00256447029134 0.00309127644105 0.00309127644105]
      | sbobj.Groups.TimeRange = [0 8.6]
  Signal 1 : Outport  Tag=STV Outport
  wires:
  Demux/1 -> Signal 1/1
  FromWs/1 -> Demux/1

== system steering_mpc/Yaw traj ==
  Demux : Demux  Tag=STV Demux  Outputs=1
      settings: DisplayOption=none
  FromWs : FromWorkspace  Tag=STV FromWs  VariableName=tuvar
      SigBuilderData=|
      | common.afterFinalStr = 'Extrapolate'
      | common.sampleTime = 0
      | dataSet.timeRange = [0 84.64]
      | dataSet.name = 'Group 1'
      | sbobj.Groups.Name = 'Group 1'
      | sbobj.Groups.Signals.Name = 'Signal 1'
      | sbobj.Groups.Signals.XData = [0 0.23 0.46 0.69 0.92 1.15 1.38 1.61 1.84 2.07 2.3 2.53 ... (369 elements, 1x369)]
      | sbobj.Groups.Signals.YData = [0 0.00105 0.005 0.008 0.012 0.014 0.018 0.0217837388916 0.0219289685923 0.0211415307273 0.0206625240453 0.0200900486735 ... (369 elements, 1x369)]
      | sbobj.Groups.TimeRange = [0 84.64]
  Signal 1 : Outport  Tag=STV Outport
  wires:
  Demux/1 -> Signal 1/1
  FromWs/1 -> Demux/1
